simulink model "Linearized Model"  (R2023b)
settings: Solver=FixedStepAuto  StartTime=0.0  StopTime=1000  FixedStep=1e-2  RelTol=1e-3
InitFcn:
  | run('init.m');
undefined symbols (not defined in the file): A, B, CC, DiscIntNeverNeededParam, U0, X0, X_prime0
libraries: slpidlib x4, simulink x1
settings Model: Creator=Marvin  LastModifiedBy=刘宸鸣

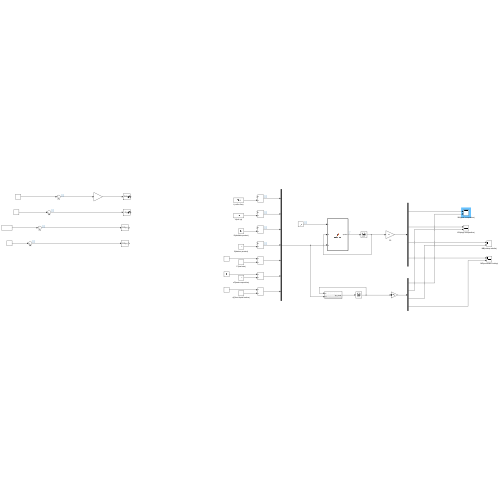
[thumbnail: Simulink's stored preview of the top-level diagram]
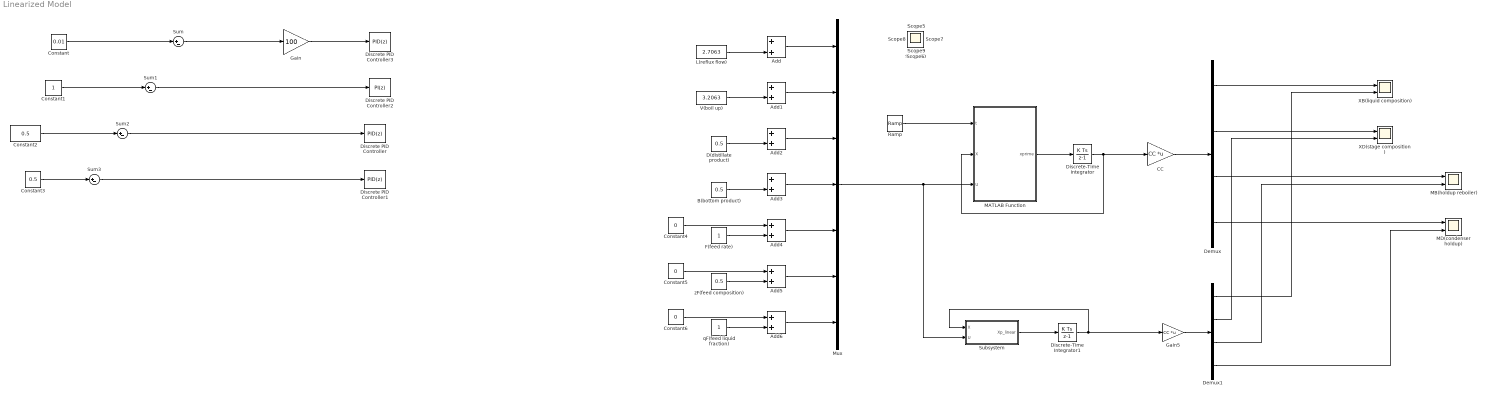
== system Linearized Model ==
  Add{,1..6} (7 alike) : Sum
  B(bottom product) : Constant  Value=0.5
  CC : Gain  Gain=CC  Multiplication=Matrix(K*u)
  Constant : Constant  Value=0.01
  Constant1 : Constant
  Constant2 : Constant  Value=0.5
  Constant3 : Constant  Value=0.5
  Constant4 : Constant  Value=0
  Constant5 : Constant  Value=0
  Constant6 : Constant  Value=0
  D(distillate product) : Constant  Value=0.5
  Demux : Demux
  Demux1 : Demux
  Discrete PID Controller : slpidlib/PID Controller  Controller=PID  Form=Parallel  TimeDomain=Discrete-time  UseExternalTs=off  SampleTime=-1  IntegratorMethod=Forward Euler  FilterMethod=Forward Euler  ControllerParametersSource=internal  P=-0.983157950111163  I=-0.192890509749347  UseKiTs=off  D=-0.00491096748781209  N=125.5780537129  UseFilter=off  TunerSelectOption=Transfer Function Based (PID Tuner App)  InitialConditionSource=internal  InitialConditionForIntegrator=0  InitialConditionForFilter=0  DifferentiatorICPrevScaledInput=0  ExternalReset=none  TrackingMode=off  Kt=1  LimitOutput=off  SatLimitsSource=internal  UpperSaturationLimit=inf  LowerSaturationLimit=-inf  LinearizeAsGain=off  AntiWindupMode=none  Kb=1  LimitIntegrator=off  UpperIntegratorSaturationLimit=inf  LowerIntegratorSaturationLimit=-inf  POutMin=[]  POutMax=[]  IOutMin=[]  IOutMax=[]  DOutMin=[]  DOutMax=[]  NOutMin=[]  NOutMax=[]  SumOutMin=[]  SumOutMax=[]  SaturationOutMin=[]  SaturationOutMax=[]  PParamMin=[]  PParamMax=[]  IParamMin=[]  IParamMax=[]  DParamMin=[]  DParamMax=[]  NParamMin=[]  NParamMax=[]  KbParamMin=[]  KbParamMax=[]  KtParamMin=[]  KtParamMax=[]  KbOutMin=[]  KbOutMax=[]  KtOutMin=[]  KtOutMax=[]  IntegratorOutMin=[]  IntegratorOutMax=[]  FilterOutMin=[]  FilterOutMax=[]  SumI1OutMin=[]  SumI1OutMax=[]  SumI2OutMin=[]  SumI2OutMax=[]  SumI3OutMin=[]  SumI3OutMax=[]  SumI4OutMin=[]  SumI4OutMax=[]  SumDOutMin=[]  SumDOutMax=[]  DifferentiatorOutMin=[]  DifferentiatorOutMax=[]  FilterDiffOutCoefMin=[]  FilterDiffOutCoefMax=[]  ReciprocalOutMin=[]  ReciprocalOutMax=[]  SumDenOutMin=[]  SumDenOutMax=[]  SumNumOutMin=[]  SumNumOutMax=[]  DivideOutMin=[]  DivideOutMax=[]  UdiffTsProdOutMin=[]  UdiffTsProdOutMax=[]  NTsProdOutMin=[]  NTsProdOutMax=[]  UintegralTsProdOutMin=[]  UintegralTsProdOutMax=[]  UngainTsProdOutMin=[]  UngainTsProdOutMax=[]  ClampingZeroOutDataTypeStr=Inherit: Inherit via back propagation  ClampingZeroOutMin=[]  ClampingZeroOutMax=[]  FilterDenConstantOutDataTypeStr=Inherit: Inherit via back propagation  FilterDenConstantOutMin=[]  FilterDenConstantOutMax=[]  PCopyOutDataTypeStr=Inherit: Inherit via back propagation  PCopyOutMin=[]  PCopyOutMax=[]  NCopyOutDataTypeStr=Inherit: Inherit via back propagation  NCopyOutMin=[]  NCopyOutMax=[]  IntegratorContinuousStateAttributes=''  IntegratorStateMustResolveToSignalObject=off  IntegratorRTWStateStorageClass=Auto  FilterContinuousStateAttributes=''  FilterStateMustResolveToSignalObject=off  FilterRTWStateStorageClass=Auto  ParallelPVariant=InternalParameters  IdealPVariant=Disabled  IVariant=InternalParameters  DVariant=InternalParameters  IntegratorVariant=Discrete  SatVariant=Disabled  AWVariant=Passthrough  PCopyVariant=Disabled  TRVariant=Disabled  FdbkBlocksVariant=Forward  IdealPFdbkVariant=Disabled  SatFdbkVariant=Disabled  DerivativeFilterVariant=Differentiator  NVariant=Passthrough  NCopyVariant=Disabled_SignalSpec  FilterICVariant=InternalICsDifferentiator  IntegratorICVariant=InternalICs  ExternalResetVariant=Disabled  TRSumVariant=Passthrough  SumFdbkVariant=Disabled  SumVariant=Sum_PID  TsampFilterVariant=InternalTs  TsampNgainVariant=Passthrough  TsampIntegralVariant=Disabled_SignalSpec  ExternalSaturationOutDataTypeStr=Inherit: Same as second input
      settings: LibrarySourceBlock=simulink/Discrete/Discrete PID Controller
  Discrete PID Controller1 : slpidlib/PID Controller  Controller=PID  Form=Parallel  TimeDomain=Discrete-time  UseExternalTs=off  SampleTime=-1  IntegratorMethod=Forward Euler  FilterMethod=Forward Euler  ControllerParametersSource=internal  P=-1.02788605439713  I=-0.196218757139595  UseKiTs=off  D=0.210779569317887  N=1.70578345077793  UseFilter=on  TunerSelectOption=Transfer Function Based (PID Tuner App)  InitialConditionSource=internal  InitialConditionForIntegrator=0  InitialConditionForFilter=0  DifferentiatorICPrevScaledInput=0  ExternalReset=none  TrackingMode=off  Kt=1  LimitOutput=off  SatLimitsSource=internal  UpperSaturationLimit=inf  LowerSaturationLimit=-inf  LinearizeAsGain=off  AntiWindupMode=none  Kb=1  LimitIntegrator=off  UpperIntegratorSaturationLimit=inf  LowerIntegratorSaturationLimit=-inf  POutMin=[]  POutMax=[]  IOutMin=[]  IOutMax=[]  DOutMin=[]  DOutMax=[]  NOutMin=[]  NOutMax=[]  SumOutMin=[]  SumOutMax=[]  SaturationOutMin=[]  SaturationOutMax=[]  PParamMin=[]  PParamMax=[]  IParamMin=[]  IParamMax=[]  DParamMin=[]  DParamMax=[]  NParamMin=[]  NParamMax=[]  KbParamMin=[]  KbParamMax=[]  KtParamMin=[]  KtParamMax=[]  KbOutMin=[]  KbOutMax=[]  KtOutMin=[]  KtOutMax=[]  IntegratorOutMin=[]  IntegratorOutMax=[]  FilterOutMin=[]  FilterOutMax=[]  SumI1OutMin=[]  SumI1OutMax=[]  SumI2OutMin=[]  SumI2OutMax=[]  SumI3OutMin=[]  SumI3OutMax=[]  SumI4OutMin=[]  SumI4OutMax=[]  SumDOutMin=[]  SumDOutMax=[]  DifferentiatorOutMin=[]  DifferentiatorOutMax=[]  FilterDiffOutCoefMin=[]  FilterDiffOutCoefMax=[]  ReciprocalOutMin=[]  ReciprocalOutMax=[]  SumDenOutMin=[]  SumDenOutMax=[]  SumNumOutMin=[]  SumNumOutMax=[]  DivideOutMin=[]  DivideOutMax=[]  UdiffTsProdOutMin=[]  UdiffTsProdOutMax=[]  NTsProdOutMin=[]  NTsProdOutMax=[]  UintegralTsProdOutMin=[]  UintegralTsProdOutMax=[]  UngainTsProdOutMin=[]  UngainTsProdOutMax=[]  ClampingZeroOutDataTypeStr=Inherit: Inherit via back propagation  ClampingZeroOutMin=[]  ClampingZeroOutMax=[]  FilterDenConstantOutDataTypeStr=Inherit: Inherit via back propagation  FilterDenConstantOutMin=[]  FilterDenConstantOutMax=[]  PCopyOutDataTypeStr=Inherit: Inherit via back propagation  PCopyOutMin=[]  PCopyOutMax=[]  NCopyOutDataTypeStr=Inherit: Inherit via back propagation  NCopyOutMin=[]  NCopyOutMax=[]  IntegratorContinuousStateAttributes=''  IntegratorStateMustResolveToSignalObject=off  IntegratorRTWStateStorageClass=Auto  FilterContinuousStateAttributes=''  FilterStateMustResolveToSignalObject=off  FilterRTWStateStorageClass=Auto  ParallelPVariant=InternalParameters  IdealPVariant=Disabled  IVariant=InternalParameters  DVariant=InternalParameters  IntegratorVariant=Discrete  SatVariant=Disabled  AWVariant=Passthrough  PCopyVariant=Disabled  TRVariant=Disabled  FdbkBlocksVariant=Forward  IdealPFdbkVariant=Disabled  SatFdbkVariant=Disabled  DerivativeFilterVariant=ForwardEulerFilter  NVariant=InternalParameters  NCopyVariant=Disabled  FilterICVariant=InternalICsFilter  IntegratorICVariant=InternalICs  ExternalResetVariant=Disabled  TRSumVariant=Passthrough  SumFdbkVariant=Disabled  SumVariant=Sum_PID  TsampFilterVariant=InternalTs  TsampNgainVariant=Passthrough  TsampIntegralVariant=Disabled_SignalSpec  ExternalSaturationOutDataTypeStr=Inherit: Same as second input
      settings: LibrarySourceBlock=simulink/Discrete/Discrete PID Controller
  Discrete PID Controller2 : slpidlib/PID Controller  Controller=PI  Form=Parallel  TimeDomain=Discrete-time  UseExternalTs=off  SampleTime=-1  IntegratorMethod=Forward Euler  FilterMethod=Forward Euler  ControllerParametersSource=internal  P=0  I=0.005  UseKiTs=off  D=3.38680797399408e-07  N=0.0956027333022247  UseFilter=off  TunerSelectOption=Transfer Function Based (PID Tuner App)  InitialConditionSource=internal  InitialConditionForIntegrator=0  InitialConditionForFilter=0  DifferentiatorICPrevScaledInput=0  ExternalReset=none  TrackingMode=off  Kt=1  LimitOutput=on  SatLimitsSource=internal  UpperSaturationLimit=5  LowerSaturationLimit=-5  LinearizeAsGain=off  AntiWindupMode=none  Kb=1  LimitIntegrator=off  UpperIntegratorSaturationLimit=inf  LowerIntegratorSaturationLimit=-inf  POutMin=[]  POutMax=[]  IOutMin=[]  IOutMax=[]  DOutMin=[]  DOutMax=[]  NOutMin=[]  NOutMax=[]  SumOutMin=[]  SumOutMax=[]  SaturationOutMin=[]  SaturationOutMax=[]  PParamMin=[]  PParamMax=[]  IParamMin=[]  IParamMax=[]  DParamMin=[]  DParamMax=[]  NParamMin=[]  NParamMax=[]  KbParamMin=[]  KbParamMax=[]  KtParamMin=[]  KtParamMax=[]  KbOutMin=[]  KbOutMax=[]  KtOutMin=[]  KtOutMax=[]  IntegratorOutMin=[]  IntegratorOutMax=[]  FilterOutMin=[]  FilterOutMax=[]  SumI1OutMin=[]  SumI1OutMax=[]  SumI2OutMin=[]  SumI2OutMax=[]  SumI3OutMin=[]  SumI3OutMax=[]  SumI4OutMin=[]  SumI4OutMax=[]  SumDOutMin=[]  SumDOutMax=[]  DifferentiatorOutMin=[]  DifferentiatorOutMax=[]  FilterDiffOutCoefMin=[]  FilterDiffOutCoefMax=[]  ReciprocalOutMin=[]  ReciprocalOutMax=[]  SumDenOutMin=[]  SumDenOutMax=[]  SumNumOutMin=[]  SumNumOutMax=[]  DivideOutMin=[]  DivideOutMax=[]  UdiffTsProdOutMin=[]  UdiffTsProdOutMax=[]  NTsProdOutMin=[]  NTsProdOutMax=[]  UintegralTsProdOutMin=[]  UintegralTsProdOutMax=[]  UngainTsProdOutMin=[]  UngainTsProdOutMax=[]  ClampingZeroOutDataTypeStr=Inherit: Inherit via back propagation  ClampingZeroOutMin=[]  ClampingZeroOutMax=[]  FilterDenConstantOutDataTypeStr=Inherit: Inherit via back propagation  FilterDenConstantOutMin=[]  FilterDenConstantOutMax=[]  PCopyOutDataTypeStr=Inherit: Inherit via back propagation  PCopyOutMin=[]  PCopyOutMax=[]  NCopyOutDataTypeStr=Inherit: Inherit via back propagation  NCopyOutMin=[]  NCopyOutMax=[]  IntegratorContinuousStateAttributes=''  IntegratorStateMustResolveToSignalObject=off  IntegratorRTWStateStorageClass=Auto  FilterContinuousStateAttributes=''  FilterStateMustResolveToSignalObject=off  FilterRTWStateStorageClass=Auto  ParallelPVariant=InternalParameters  IdealPVariant=Disabled  IVariant=InternalParameters  DVariant=Disabled  IntegratorVariant=Discrete  SatVariant=Enabled  AWVariant=Passthrough  PCopyVariant=Disabled  TRVariant=Disabled  FdbkBlocksVariant=Forward  IdealPFdbkVariant=Disabled  SatFdbkVariant=Disabled  DerivativeFilterVariant=Disabled  NVariant=Disabled  NCopyVariant=Disabled_SignalSpec  FilterICVariant=Disabled  IntegratorICVariant=InternalICs  ExternalResetVariant=Disabled  TRSumVariant=Passthrough  SumFdbkVariant=Disabled  SumVariant=Sum_PI  TsampFilterVariant=InternalTs  TsampNgainVariant=Passthrough  TsampIntegralVariant=Disabled_SignalSpec  ExternalSaturationOutDataTypeStr=Inherit: Same as second input
      settings: LibrarySourceBlock=simulink/Discrete/Discrete PID Controller
  Discrete PID Controller3 : slpidlib/PID Controller  Controller=PID  Form=Parallel  TimeDomain=Discrete-time  UseExternalTs=off  SampleTime=-1  IntegratorMethod=Forward Euler  FilterMethod=Forward Euler  ControllerParametersSource=internal  P=0.0244843541929658  I=0.000251904441952452  UseKiTs=off  D=0.000122415473353791  N=24.0722804363654  UseFilter=off  TunerSelectOption=Transfer Function Based (PID Tuner App)  InitialConditionSource=internal  InitialConditionForIntegrator=0  InitialConditionForFilter=0  DifferentiatorICPrevScaledInput=0  ExternalReset=none  TrackingMode=off  Kt=1  LimitOutput=on  SatLimitsSource=internal  UpperSaturationLimit=5  LowerSaturationLimit=-5  LinearizeAsGain=off  AntiWindupMode=none  Kb=1  LimitIntegrator=off  UpperIntegratorSaturationLimit=inf  LowerIntegratorSaturationLimit=-inf  POutMin=[]  POutMax=[]  IOutMin=[]  IOutMax=[]  DOutMin=[]  DOutMax=[]  NOutMin=[]  NOutMax=[]  SumOutMin=[]  SumOutMax=[]  SaturationOutMin=[]  SaturationOutMax=[]  PParamMin=[]  PParamMax=[]  IParamMin=[]  IParamMax=[]  DParamMin=[]  DParamMax=[]  NParamMin=[]  NParamMax=[]  KbParamMin=[]  KbParamMax=[]  KtParamMin=[]  KtParamMax=[]  KbOutMin=[]  KbOutMax=[]  KtOutMin=[]  KtOutMax=[]  IntegratorOutMin=[]  IntegratorOutMax=[]  FilterOutMin=[]  FilterOutMax=[]  SumI1OutMin=[]  SumI1OutMax=[]  SumI2OutMin=[]  SumI2OutMax=[]  SumI3OutMin=[]  SumI3OutMax=[]  SumI4OutMin=[]  SumI4OutMax=[]  SumDOutMin=[]  SumDOutMax=[]  DifferentiatorOutMin=[]  DifferentiatorOutMax=[]  FilterDiffOutCoefMin=[]  FilterDiffOutCoefMax=[]  ReciprocalOutMin=[]  ReciprocalOutMax=[]  SumDenOutMin=[]  SumDenOutMax=[]  SumNumOutMin=[]  SumNumOutMax=[]  DivideOutMin=[]  DivideOutMax=[]  UdiffTsProdOutMin=[]  UdiffTsProdOutMax=[]  NTsProdOutMin=[]  NTsProdOutMax=[]  UintegralTsProdOutMin=[]  UintegralTsProdOutMax=[]  UngainTsProdOutMin=[]  UngainTsProdOutMax=[]  ClampingZeroOutDataTypeStr=Inherit: Inherit via back propagation  ClampingZeroOutMin=[]  ClampingZeroOutMax=[]  FilterDenConstantOutDataTypeStr=Inherit: Inherit via back propagation  FilterDenConstantOutMin=[]  FilterDenConstantOutMax=[]  PCopyOutDataTypeStr=Inherit: Inherit via back propagation  PCopyOutMin=[]  PCopyOutMax=[]  NCopyOutDataTypeStr=Inherit: Inherit via back propagation  NCopyOutMin=[]  NCopyOutMax=[]  IntegratorContinuousStateAttributes=''  IntegratorStateMustResolveToSignalObject=off  IntegratorRTWStateStorageClass=Auto  FilterContinuousStateAttributes=''  FilterStateMustResolveToSignalObject=off  FilterRTWStateStorageClass=Auto  ParallelPVariant=InternalParameters  IdealPVariant=Disabled  IVariant=InternalParameters  DVariant=InternalParameters  IntegratorVariant=Discrete  SatVariant=Enabled  AWVariant=Passthrough  PCopyVariant=Disabled  TRVariant=Disabled  FdbkBlocksVariant=Forward  IdealPFdbkVariant=Disabled  SatFdbkVariant=Disabled  DerivativeFilterVariant=Differentiator  NVariant=Passthrough  NCopyVariant=Disabled_SignalSpec  FilterICVariant=InternalICsDifferentiator  IntegratorICVariant=InternalICs  ExternalResetVariant=Disabled  TRSumVariant=Passthrough  SumFdbkVariant=Disabled  SumVariant=Sum_PID  TsampFilterVariant=InternalTs  TsampNgainVariant=Passthrough  TsampIntegralVariant=Disabled_SignalSpec  ExternalSaturationOutDataTypeStr=Inherit: Same as second input
      settings: LibrarySourceBlock=simulink/Discrete/Discrete PID Controller
  Discrete-Time Integrator : DiscreteIntegrator  InitialCondition=X0  SampleTime=-1  ICPrevOutput=DiscIntNeverNeededParam  ICPrevScaledInput=DiscIntNeverNeededParam
  Discrete-Time Integrator1 : DiscreteIntegrator  InitialCondition=X0  SampleTime=-1  ICPrevOutput=DiscIntNeverNeededParam  ICPrevScaledInput=DiscIntNeverNeededParam
  F(feed rate) : Constant
  Gain : Gain  Gain=100
  Gain5 : Gain  Gain=CC  Multiplication=Matrix(K*u)
  L(reflux flow) : Constant  Value=2.7063
  MATLAB Function : MATLAB Function  TreatAsAtomicUnit=on
  MB(holdup reboiler) : Scope  NumInputPorts=2
  MD(condenser holdup) : Scope  NumInputPorts=2
  Mux : Mux  Inputs=7
  Ramp : simulink/Sources/Ramp  slope=1  start=0  InitialOutput=0
  Subsystem : Subsystem
  Sum{,1..3} (4 alike) : Sum  Inputs=|+-
  V(boil up) : Constant  Value=3.2063
  XB(liquid composition) : Scope  NumInputPorts=2
  XD(stage composition) : Scope  NumInputPorts=2
  qF(feed liquid fraction) : Constant
  zF(feed composition) : Constant  Value=0.5
  Scope{,1..10} (11 alike) : Scope
  wires:
  Ramp/1 -> MATLAB Function/1(t)
  MATLAB Function/1(xprime) -> Discrete-Time Integrator/1
  Discrete-Time Integrator/1 -> MATLAB Function/2(X), CC/1
  CC/1 -> Demux/1
  Demux/3 -> MB(holdup reboiler)/1
  Demux/2 -> XD(stage composition)/1
  Constant/1 -> Sum/1
  Add1/1 -> Mux/2
  Sum1/1 -> Discrete PID Controller2/1
  Constant1/1 -> Sum1/1
  Add2/1 -> Mux/3
  Constant2/1 -> Sum2/1
  Add3/1 -> Mux/4
  Sum3/1 -> Discrete PID Controller1/1
  Constant3/1 -> Sum3/1
  Add4/1 -> Mux/5
  F(feed rate)/1 -> Add4/2
  Constant4/1 -> Add4/1
  Add5/1 -> Mux/6
  zF(feed composition)/1 -> Add5/2
  Constant5/1 -> Add5/1
  Add6/1 -> Mux/7
  qF(feed liquid fraction)/1 -> Add6/2
  Constant6/1 -> Add6/1
  L(reflux flow)/1 -> Add/2
  V(boil up)/1 -> Add1/2
  D(distillate product)/1 -> Add2/2
  B(bottom product)/1 -> Add3/2
  Sum2/1 -> Discrete PID Controller/1
  Demux/1 -> XB(liquid composition)/1
  Demux/4 -> MD(condenser holdup)/1
  Sum/1 -> Gain/1
  Add/1 -> Mux/1
  Gain/1 -> Discrete PID Controller3/1
  Mux/1 -> Subsystem/2(U), MATLAB Function/3(U)
  Gain5/1 -> Demux1/1
  Subsystem/1(Xp_linear) -> Discrete-Time Integrator1/1
  Discrete-Time Integrator1/1 -> Subsystem/1(X), Gain5/1
  Demux1/2 -> XD(stage composition)/2
  Demux1/3 -> MB(holdup reboiler)/2
  Demux1/4 -> MD(condenser holdup)/2
  Demux1/1 -> XB(liquid composition)/2

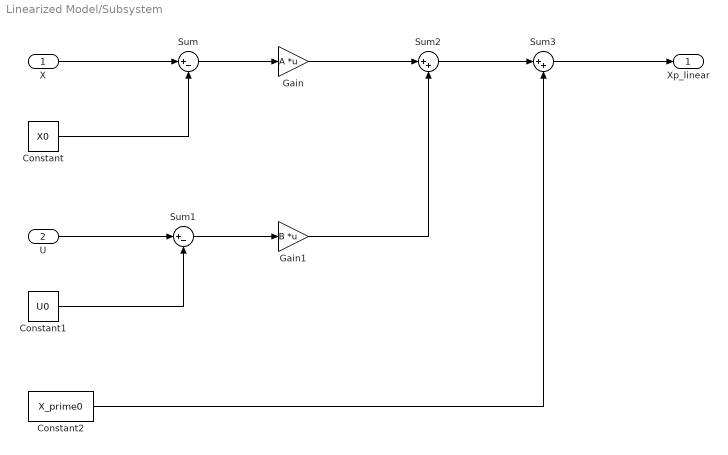
== system Linearized Model/Subsystem ==
  X : Inport
  U : Inport  Port=2
  Constant : Constant  Value=X0
  Constant1 : Constant  Value=U0
  Constant2 : Constant  Value=X_prime0
  Gain : Gain  Gain=A  Multiplication=Matrix(K*u)
  Gain1 : Gain  Gain=B  Multiplication=Matrix(K*u)
  Sum : Sum  Inputs=|+-
  Sum1 : Sum  Inputs=|+-
  Sum2 : Sum  Inputs=|++
  Sum3 : Sum  Inputs=|++
  Xp_linear : Outport
  wires:
  X/1 -> Sum/1
  Constant/1 -> Sum/2
  U/1 -> Sum1/1
  Constant1/1 -> Sum1/2
  Sum/1 -> Gain/1
  Sum1/1 -> Gain1/1
  Gain/1 -> Sum2/1
  Gain1/1 -> Sum2/2
  Sum2/1 -> Sum3/1
  Constant2/1 -> Sum3/2
  Sum3/1 -> Xp_linear/1

== matlab function Linearized Model/MATLAB Function ==
  data: t input; xprime output; X input; U input
function xprime=colamod(t,X,U)
%
% colamod - This is a nonlinear model of a distillation column with
%           NT-1 theoretical stages including a reboiler (stage 1) plus a
%           total condenser ("stage" NT). The liquid flow dynamics are
%           modelled by a simple linear relationship.
%           Model assumptions: Two components (binary separation); constant
%           relative volatility; no vapor holdup; one feed and two products;
%           constant molar flows (same vapor flow on all stages);
%           total condenser
%
%           The model is based on column A in Skogestad and Postlethwaite
%           (1996). The model has 82 states.
%
% Inputs:    t    - time in [min].
%            X    - State, the first 41 states are compositions of light
%                   component A with reboiler/bottom stage as X(1) and
%                   condenser as X(41). State X(42)is holdup in reboiler/
%                   bottom stage and X(82) is hold-up in condenser.
%            U(1) - reflux L,
%            U(2) - boilup V,
%            U(3) - top or distillate product flow D,
%            U(4) - bottom product flow B,
%            U(5) - feed rate F,
%            U(6) - feed composition, zF.
%            U(7) - feed liquid fraction, qF.
%
% Outputs:   xprime - vector with time derivative of all the states
%%%%%%%%%%%%%%%%%%%%%%%%%%%%%%%%%%%%%%%%%%%%%%%%%%%%%%%%%

%------------------------------------------------------------
% The following data need to be changed for a new column.
% These data are for "colmn A".
% Number of stages (including reboiler and total condenser:
NT=41;
% Location of feed stage (stages are counted from the bottom):
NF=21;
% Relative volatility
alpha=1.5;
% Nominal liquid holdups
M0 = zeros(1,NT);
M0(1)=0.5;      	% Nominal reboiler holdup (kmol)
i=2:NT-1; M0(i)=0.5*ones(1,NT-2);% Nominal stage (tray) holdups (kmol)
M0(NT)=0.5;      	% Nominal condenser holdup (kmol)
% Data for linearized liquid flow dynamics (does not apply to reboiler and condenser):
taul=0.063;     	% time constant for liquid dynamics (min)
F0=1;	 	% Nominal feed rate (kmol/min)
qF0 = 1; 		% Nominal fraction of liquid in feed
L0=2.70629;     	% Nominal reflux flow (from steady-state data)
L0b=L0 + qF0*F0;	% Nominal liquid flow below feed (kmol/min)
lambda=0;		% Effect of vapor flow on liquid flow ("K2-effect")
V0=3.20629;V0t=V0+(1-qF0)*F0;% Nominal vapor flows - only needed if lambda is nonzero
% End data which need to be changed
%------------------------------------------------------------

% Splitting the states
x=X(1:NT)';                          % Liquid composition from btm to top
M=X(NT+1:2*NT)';                     % Liquid hold up from btm to top

% Inputs and disturbances
LT = U(1);                            % Reflux
VB = U(2);                            % Boilup
D  = U(3);                            % Distillate
B  = U(4);                            % Bottoms

F  = U(5);                            % Feedrate
zF = U(6);                            % Feed composition
qF = U(7);                            % Feed liquid fraction

% THE MODEL

y = zeros(1,NT);
% Vapor-liquid equilibria
for i=1:1:NT-1
    y(i)=alpha*x(i)./(1+(alpha-1)*x(i));
end

% Vapor Flows assuming constant molar flows

V = VB*ones(1,NT-1);

for i=NF:1:NT-1
    V(i)=V(i) + (1-qF)*F;
end

% Liquid flows assuming linearized tray hydraulics with time constant taul
% Also includes coefficient lambda for effect of vapor flow ("K2-effect").
L = zeros(1,NT);
for i=2:1:NF
    L(i) = L0b + (M(i)-M0(i))./taul + lambda.*(V(i-1)-V0);
end

for i=NF+1:1:NT-1
L(i) = L0  + (M(i)-M0(i))./taul + lambda.*(V(i-1)-V0t);
end



L(NT)=LT;

% Time derivatives from  material balances for
% 1) total holdup and 2) component holdup

% Column
dMdt = zeros(1,NT);
dMxdt = zeros(1,NT);
for i=2:1:NT-1
dMdt(i) = L(i+1)         - L(i)       + V(i-1)         - V(i);
dMxdt(i)= L(i+1).*x(i+1) - L(i).*x(i) + V(i-1).*y(i-1) - V(i).*y(i);
end
% Correction for feed at the feed stage
% The feed is assumed to be mixed into the feed stage
dMdt(NF) = dMdt(NF)  + F;
dMxdt(NF)= dMxdt(NF) + F*zF;

% Reboiler (assumed to be an equilibrium stage)
dMdt(1) = L(2)      - V(1)      - B;
dMxdt(1)= L(2)*x(2) - V(1)*y(1) - B*x(1);

% Total condenser (no equilibrium stage)
dMdt(NT) = V(NT-1)         - LT       - D;
dMxdt(NT)= V(NT-1)*y(NT-1) - LT*x(NT) - D*x(NT);

% Compute the derivative for the mole fractions from d(Mx) = x dM + M dx
dxdt = zeros(1,NT);
for i=1:1:NT
dxdt(i) = (dMxdt(i) - x(i).*dMdt(i) )./M(i);
end

% Output
xprime=[dxdt';dMdt'];

end
